simulink model "rov_openloop"  (Simulink 6.0)
settings: Solver=ode45  StartTime=0.0  StopTime=500  RelTol=1e-3
values from neighbouring files (symbols this model uses):
  B = 53400    [npsauv.m]
  Kpdot = -1.0e-3    (= -0.001)    [npsauv.m]
  m = 5454.54/(rho/2*L^3)    (= 0.0732757914251)    [npsauv.m]
  M = r3*(Muw*u*w + Mvv*v^2) +     r4*(Muq*u*q + Mvp*v*p + Mvr*v*r) +     r5*(Mpp*p^2 + Mpr*p*r + Mrr*r^2) -      (xG*W-xB*B)*c1*c2 - (zG*W-zB*B)*s2 +      (Iz-Ix)*p*r + Ixy*q*r - Iyz*p*q - (p^2-r^2)*Ixz +      m*(rho/2*L^3)*(xG*(v*p-u*q) - zG*(w*q-v*r)) + tau5 - rho/2*Cm    [npsauv.m]
  Mqdot = -1.7e-2    (= -0.017)    [npsauv.m]
  Nrdot = -3.4e-3    (= -0.0034)    [npsauv.m]
  W = 53400    [npsauv.m]
  Xudot = -7.6e-3    (= -0.0076)    [npsauv.m]
  Yvdot = -5.5e-2    (= -0.055)    [npsauv.m]
  Zwdot = -2.4e-1    (= -0.24)    [npsauv.m]
undefined symbols (not defined in the file or in its folder): DL, DQ, I, Ma, rg, T, xb, xg, yb, yg, zb, zg
libraries: simulink x8
CloseFcn:
  | rtwprivate ssgensfun ModelCloseRequest openloop
settings Model: LastModifiedBy=c chin

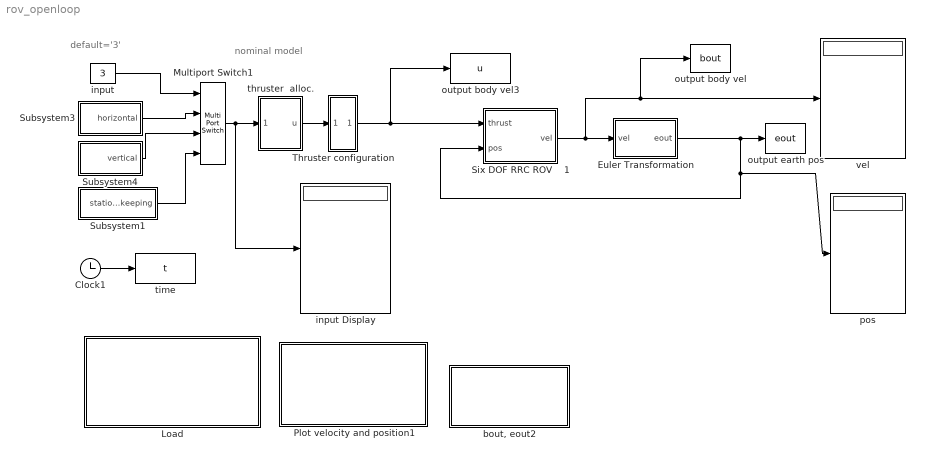
== system rov_openloop ==
  note: nominal model
  note: default='3'
  " Load  " : Subsystem
      settings: OpenFcn=|
      | clc
      | cd c:\Matlab7\toolbox\rov_design_analysis\\mat_file ;
      | load rrcrovf;
      mask Display: disp('Double-click \n to \n Load the\n RRCROV\n parameters')
  " Six DOF RRC ROV    1" : Subsystem
      mask Display:
      | disp('ROV')
      | image(imread('/rov_design_analysis/fig/ROVRRC2.jpg'));
      | color('black');port_label('input',1,'thrust')
      | color('black');port_label('input',2,'pos')
      | color('black');port_label('output',1,'vel')
      | color('black');port_label('output',2,'Inv_MC')
  Clock1 : Clock
      settings: Decimation=10
  Euler Transformation : Subsystem  AncestorBlock=rov_design_analysis/Scope Utilities/Euler Transformation
  Multiport Switch1 : MultiPortSwitch  Inputs=3
  Plot velocity and position1 : Subsystem
      settings: OpenFcn=|
      | clc
      | cd c:\Matlab7\toolbox\rov_design_analysis\\m_file ;
      | run nonlin_resp6
      mask Display: disp('Double-click \n to \n Plot Velocity \n and \n Position')
  Subsystem1 : Subsystem
  Subsystem3 : Subsystem
  Subsystem4 : Subsystem
  Thruster configuration : Subsystem
      mask Display: disp('T')
  "bout, eout2" : Subsystem
      settings: OpenFcn=|
      | clc
      | cd c:\Matlab7\toolbox\rov_design_analysis\\m_file ;
      | figure
      | plot3(eout(:,1), eout(:,2),-eout(:,3))
      | xlabel('x')
      | ylabel('y')
      | zlabel('z')
      | grid on
      mask Display: disp('Plot \n 3D Response')
  input Display : Display
  "input " : Constant  Value=3
  output body vel : ToWorkspace  VariableName=bout  SampleTime=1  SaveFormat=Array
  output body vel3 : ToWorkspace  VariableName=u  SampleTime=1  SaveFormat=Array
  output earth pos : ToWorkspace  VariableName=eout  SampleTime=1  SaveFormat=Array
  pos : Display
  "thruster  alloc.  " : Subsystem
  time : ToWorkspace  VariableName=t  SampleTime=1  SaveFormat=Array
  vel : Display
  wires:
  Thruster configuration/1(output force) -> output body vel3/1, " Six DOF RRC ROV    1"/1("thrust ")
  Clock1/1 -> time/1
  Subsystem4/1(vertical) -> Multiport Switch1/3
  Subsystem3/1(horizontal) -> Multiport Switch1/2
  "input "/1 -> Multiport Switch1/1
  Subsystem1/1(station-keeping) -> Multiport Switch1/4
  Multiport Switch1/1 -> "thruster  alloc.  "/1(ubar_i), input Display/1
  "thruster  alloc.  "/1(u) -> Thruster configuration/1(input velocity)
  Euler Transformation/1(eout) -> output earth pos/1, pos/1, " Six DOF RRC ROV    1"/2("pos ")
  " Six DOF RRC ROV    1"/1(vel) -> Euler Transformation/1(vel), output body vel/1, vel/1

== system rov_openloop/ Load   ==

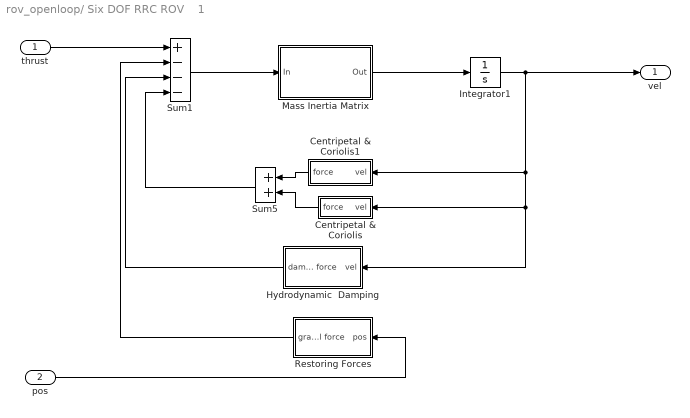
== system rov_openloop/ Six DOF RRC ROV    1 ==
  "thrust " : Inport  Port=1  LatchInput=off
  "pos " : Inport  Port=2  LatchInput=off
  Centripetal & Coriolis : Subsystem  Orientation=left  AncestorBlock=rov_design_analysis/ROV Models/1. Six DOF RRC ROV II/Centripetal & Coriolis
      mask Display: disp('C')
  Centripetal & Coriolis1 : Subsystem  Orientation=left
      mask Display: disp('CA')
  Hydrodynamic  Damping : Subsystem  Orientation=left
      mask Display: disp('Hydrodynamic \nDamping')
  Integrator1 : Integrator
  Mass Inertia Matrix : Subsystem
      mask Display: disp('inv(MRB+MA)')
  Restoring Forces : Subsystem  Orientation=left
      mask Display: disp('Restoring\nForce')
  Sum1 : Sum  Inputs=+---  SaturateOnIntegerOverflow=on  InputSameDT=on
  Sum5 : Sum  Orientation=left  SaturateOnIntegerOverflow=on  InputSameDT=on
  vel : Outport
  wires:
  Restoring Forces/1(gravitational force) -> Sum1/2
  Hydrodynamic  Damping/1(damping force) -> Sum1/3
  "thrust "/1 -> Sum1/1
  Sum1/1 -> Mass Inertia Matrix/1(In)
  Integrator1/1 -> vel/1, Centripetal & Coriolis/1(vel), Hydrodynamic  Damping/1(vel), Centripetal & Coriolis1/1(vel)
  "pos "/1 -> Restoring Forces/1(pos)
  Mass Inertia Matrix/1(Out) -> Integrator1/1
  Centripetal & Coriolis1/1(force) -> Sum5/1
  Centripetal & Coriolis/1(force) -> Sum5/2
  Sum5/1 -> Sum1/4

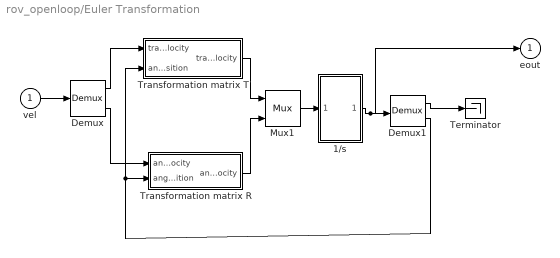
== system rov_openloop/Euler Transformation ==
  vel : Inport  Port=1  LatchInput=off
  1/s : Subsystem
  Demux : Demux  Outputs=2
  Demux1 : Demux  Outputs=2
  Mux1 : Mux  Inputs=2
  Terminator : Terminator
  Transformation matrix R : Subsystem
      mask Display: disp('Transformation R')
  Transformation matrix T : Subsystem
      mask Display: disp('Transformation T')
  eout : Outport  InitialOutput=0
  wires:
  Mux1/1 -> 1/s/1(In1)
  1/s/1(Out1) -> Demux1/1, eout/1
  Demux/2 -> Transformation matrix R/1(angular body  velocity)
  Demux/1 -> Transformation matrix T/1(translational body velocity)
  vel/1 -> Demux/1
  Demux1/2 -> Transformation matrix T/2(angular position), Transformation matrix R/2(angular position)
  Transformation matrix R/1(angular earth velocity) -> Mux1/2
  Transformation matrix T/1(translational earth velocity) -> Mux1/1
  Demux1/1 -> Terminator/1

== system rov_openloop/Plot velocity and position1 ==

== system rov_openloop/Subsystem1 ==
  Mux1 : Mux
  uc{1..4} (4 alike) : Step  Time=0  SampleTime=0
  station-keeping : Outport
  wires:
  uc2/1 -> Mux1/2
  uc1/1 -> Mux1/1
  uc3/1 -> Mux1/3
  uc4/1 -> Mux1/4
  Mux1/1 -> station-keeping/1

== system rov_openloop/Subsystem3 ==
  Mux1 : Mux
  u1 : Step  Time=0  SampleTime=0
  u2 : Step  Time=0  SampleTime=0
  u3 : Step  Time=0  After=0  SampleTime=0
  u4 : Step  Time=0  After=0  SampleTime=0
  horizontal : Outport
  wires:
  u2/1 -> Mux1/2
  u1/1 -> Mux1/1
  u3/1 -> Mux1/3
  Mux1/1 -> horizontal/1
  u4/1 -> Mux1/4

== system rov_openloop/Subsystem4 ==
  Mux1 : Mux
  u1 : Step  Time=0  After=0  SampleTime=0
  u2 : Step  Time=0  After=0  SampleTime=0
  u3 : Step  Time=0  SampleTime=0
  u4 : Step  Time=0  SampleTime=0
  vertical : Outport
  wires:
  u2/1 -> Mux1/2
  u1/1 -> Mux1/1
  u3/1 -> Mux1/3
  u4/1 -> Mux1/4
  Mux1/1 -> vertical/1

== system rov_openloop/Thruster configuration ==
  input velocity : Inport  Orientation=up  Port=1  LatchInput=off
  Thruster Matrix : Gain  Gain=T  Multiplication=Matrix(K*u)  SaturateOnIntegerOverflow=on
  output force : Outport  InitialOutput=0
  wires:
  input velocity/1 -> Thruster Matrix/1
  Thruster Matrix/1 -> output force/1

== system rov_openloop/bout, eout2 ==

== system rov_openloop/thruster  alloc.   ==
  ubar_i : Inport  Port=1  LatchInput=off
  " input" : Constant  Value=[ 1 1 1 1]'
  thruster  allocation control1 : Subsystem  AncestorBlock=|
      | rov_design_analysis/ROV Controller
      | Design
      | Applications/1. Heading autopilot/thruster 
      | allocation control
  u : Outport
  wires:
  ubar_i/1 -> thruster  allocation control1/1(vel)
  " input"/1 -> thruster  allocation control1/2(on/off)
  thruster  allocation control1/1(volt) -> u/1

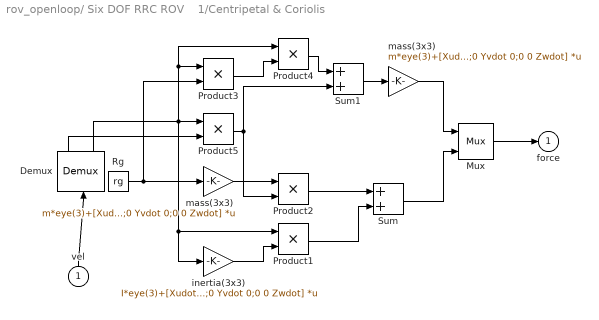
== system rov_openloop/ Six DOF RRC ROV    1/Centripetal & Coriolis ==
  vel : Inport  Orientation=up  Port=1  LatchInput=off
  Demux : Demux  Orientation=up  Outputs=2
  Mux : Mux  Inputs=2
  Product{1..5} (5 alike) : Product  SaturateOnIntegerOverflow=on  RndMeth=Zero  InputSameDT=on
  Rg : Constant  Value=rg
  Sum : Sum  SaturateOnIntegerOverflow=on  InputSameDT=on
  Sum1 : Sum  SaturateOnIntegerOverflow=on  InputSameDT=on
  inertia(3x3) : Gain  Gain=I*eye(3)+[Xudot 0 0;0 Yvdot 0;0 0 Zwdot]  Multiplication=Matrix(K*u)  SaturateOnIntegerOverflow=on
  "mass(3x3) " : Gain  Gain=m*eye(3)+[Xudot 0 0;0 Yvdot 0;0 0 Zwdot]  Multiplication=Matrix(K*u)  SaturateOnIntegerOverflow=on
  "mass(3x3)   " : Gain  Gain=m*eye(3)+[Xudot 0 0;0 Yvdot 0;0 0 Zwdot]  Multiplication=Matrix(K*u)  SaturateOnIntegerOverflow=on
  force : Outport  InitialOutput=0
  wires:
  Product1/1 -> Sum/2
  "mass(3x3)   "/1 -> Product2/1
  Product2/1 -> Sum/1
  Rg/1 -> Product3/2, "mass(3x3)   "/1
  Product3/1 -> Product4/2
  Product4/1 -> Sum1/1
  Product5/1 -> Product2/2, Sum1/2
  Sum1/1 -> "mass(3x3) "/1
  Demux/2 -> Product5/1, Product3/1, Product4/1, Product1/1, inertia(3x3)/1
  Demux/1 -> Product5/2
  vel/1 -> Demux/1
  inertia(3x3)/1 -> Product1/2
  "mass(3x3) "/1 -> Mux/1
  Sum/1 -> Mux/2
  Mux/1 -> force/1

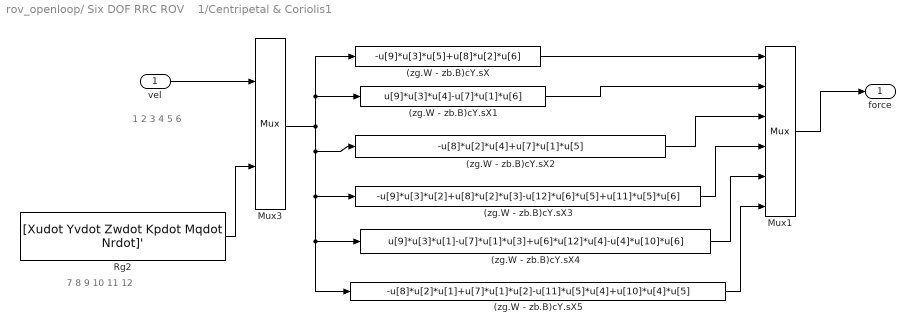
== system rov_openloop/ Six DOF RRC ROV    1/Centripetal & Coriolis1 ==
  note: 7 8 9 10 11 12
  note: 1 2 3 4 5 6
  vel : Inport  Port=1  LatchInput=off
  (zg.W - zb.B)cY.sX : Fcn  Expr=-u[9]*u[3]*u[5]+u[8]*u[2]*u[6]
  (zg.W - zb.B)cY.sX1 : Fcn  Expr=u[9]*u[3]*u[4]-u[7]*u[1]*u[6]
  (zg.W - zb.B)cY.sX2 : Fcn  Expr=-u[8]*u[2]*u[4]+u[7]*u[1]*u[5]
  (zg.W - zb.B)cY.sX3 : Fcn  Expr=-u[9]*u[3]*u[2]+u[8]*u[2]*u[3]-u[12]*u[6]*u[5]+u[11]*u[5]*u[6]
  (zg.W - zb.B)cY.sX4 : Fcn  Expr=u[9]*u[3]*u[1]-u[7]*u[1]*u[3]+u[6]*u[12]*u[4]-u[4]*u[10]*u[6]
  (zg.W - zb.B)cY.sX5 : Fcn  Expr=-u[8]*u[2]*u[1]+u[7]*u[1]*u[2]-u[11]*u[5]*u[4]+u[10]*u[4]*u[5]
  Mux1 : Mux  Inputs=6
  Mux3 : Mux  Inputs=2
  Rg2 : Constant  Value=[Xudot Yvdot Zwdot Kpdot Mqdot Nrdot]'
  force : Outport
  wires:
  Mux1/1 -> force/1
  (zg.W - zb.B)cY.sX/1 -> Mux1/1
  (zg.W - zb.B)cY.sX1/1 -> Mux1/2
  (zg.W - zb.B)cY.sX2/1 -> Mux1/3
  (zg.W - zb.B)cY.sX3/1 -> Mux1/4
  (zg.W - zb.B)cY.sX4/1 -> Mux1/5
  (zg.W - zb.B)cY.sX5/1 -> Mux1/6
  vel/1 -> Mux3/1
  Rg2/1 -> Mux3/2
  Mux3/1 -> (zg.W - zb.B)cY.sX/1, (zg.W - zb.B)cY.sX1/1, (zg.W - zb.B)cY.sX4/1, (zg.W - zb.B)cY.sX5/1, (zg.W - zb.B)cY.sX3/1, (zg.W - zb.B)cY.sX2/1

== system rov_openloop/ Six DOF RRC ROV    1/Hydrodynamic  Damping ==
  vel : Inport  Port=1  LatchInput=off
  D linear : Gain  Gain=-diag(DL)  SaturateOnIntegerOverflow=on
  D quadratic : Gain  Gain=-diag(DQ)  SaturateOnIntegerOverflow=on
  Product : Product  SaturateOnIntegerOverflow=on  RndMeth=Zero  InputSameDT=on
  Sum2 : Sum  SaturateOnIntegerOverflow=on  InputSameDT=on
  |u| : Abs  SaturateOnIntegerOverflow=on
  damping force : Outport  InitialOutput=0
  wires:
  vel/1 -> D linear/1, Product/1, |u|/1
  Product/1 -> D quadratic/1
  |u|/1 -> Product/2
  D quadratic/1 -> Sum2/1
  D linear/1 -> Sum2/2
  Sum2/1 -> damping force/1

== system rov_openloop/ Six DOF RRC ROV    1/Mass Inertia Matrix ==
  In : Inport  Port=1  LatchInput=off
  inverse M : Gain  Gain=inv(M+Ma)  Multiplication=Matrix(K*u)  SaturateOnIntegerOverflow=on
  Out : Outport
  wires:
  inverse M/1 -> Out/1
  In/1 -> inverse M/1

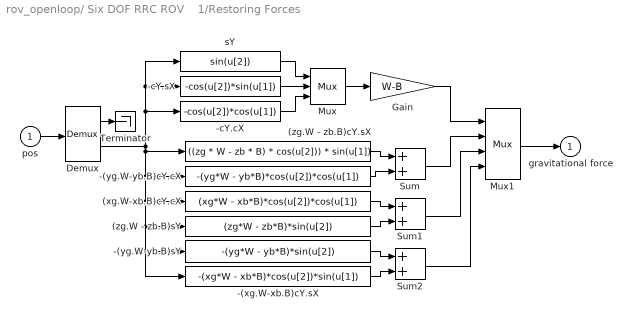
== system rov_openloop/ Six DOF RRC ROV    1/Restoring Forces ==
  pos : Inport  Port=1  LatchInput=off
  (xg.W-xb.B)cY.cX : Fcn  Expr=(xg*W - xb*B)*cos(u[2])*cos(u[1])
  (zg.W - zb.B)cY.sX : Fcn  Expr=((zg * W - zb * B) * cos(u[2])) * sin(u[1])
  (zg.W - zb.B)sY : Fcn  Expr=(zg*W - zb*B)*sin(u[2])
  -(xg.W-xb.B)cY.sX : Fcn  Expr=-(xg*W - xb*B)*cos(u[2])*sin(u[1])
  -(yg.W-yb.B)cY.cX : Fcn  Expr=-(yg*W - yb*B)*cos(u[2])*cos(u[1])
  -(yg.W-yb.B)sY : Fcn  Expr=-(yg*W - yb*B)*sin(u[2])
  -cY.cX : Fcn  Expr=-cos(u[2])*cos(u[1])
  -cY.sX : Fcn  Expr=-cos(u[2])*sin(u[1])
  Demux : Demux  Outputs=2
  Gain : Gain  Gain=W-B  SaturateOnIntegerOverflow=on
  Mux : Mux  Inputs=3
  Mux1 : Mux
  Sum : Sum  SaturateOnIntegerOverflow=on  InputSameDT=on
  Sum1 : Sum  SaturateOnIntegerOverflow=on  InputSameDT=on
  Sum2 : Sum  SaturateOnIntegerOverflow=on  InputSameDT=on
  Terminator : Terminator
  sY : Fcn  Expr=sin(u[2])
  gravitational force : Outport  InitialOutput=0
  wires:
  Sum2/1 -> Mux1/4
  -(yg.W-yb.B)sY/1 -> Sum2/1
  -(xg.W-xb.B)cY.sX/1 -> Sum2/2
  Sum1/1 -> Mux1/3
  (xg.W-xb.B)cY.cX/1 -> Sum1/1
  (zg.W - zb.B)sY/1 -> Sum1/2
  Sum/1 -> Mux1/2
  (zg.W - zb.B)cY.sX/1 -> Sum/1
  -(yg.W-yb.B)cY.cX/1 -> Sum/2
  Gain/1 -> Mux1/1
  Mux/1 -> Gain/1
  -cY.cX/1 -> Mux/3
  -cY.sX/1 -> Mux/2
  sY/1 -> Mux/1
  Mux1/1 -> gravitational force/1
  Demux/2 -> -(xg.W-xb.B)cY.sX/1, -(yg.W-yb.B)sY/1, (zg.W - zb.B)sY/1, (xg.W-xb.B)cY.cX/1, -(yg.W-yb.B)cY.cX/1, (zg.W - zb.B)cY.sX/1, sY/1, -cY.sX/1, -cY.cX/1
  Demux/1 -> Terminator/1
  pos/1 -> Demux/1

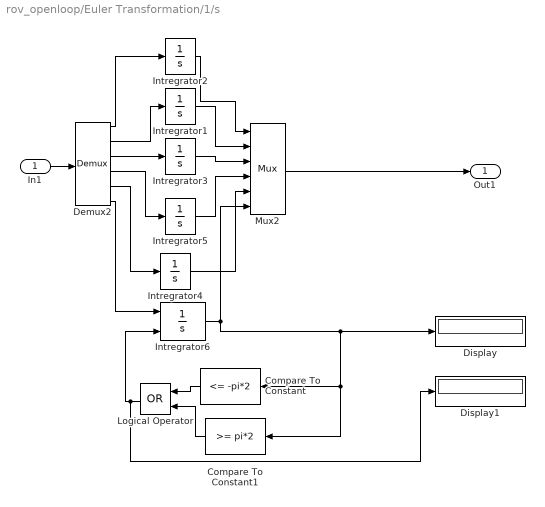
== system rov_openloop/Euler Transformation/1/s ==
  In1 : Inport  Port=1  LatchInput=off
  Compare To Constant : simulink/Logic and Bit Operations/Compare To Constant  Orientation=left  relop=<=  const=-pi*2  LogicOutDataTypeMode=boolean
  Compare To Constant1 : simulink/Logic and Bit Operations/Compare To Constant  Orientation=left  relop=>=  const=pi*2  LogicOutDataTypeMode=boolean
  Demux2 : Demux  Outputs=6
  Display : Display
  Display1 : Display
  Intregrator{1..5} (5 alike) : Integrator
  Intregrator6 : Integrator  ExternalReset=rising  InitialCondition=0.5
  Logical Operator : Logic  Orientation=left  Operator=OR  AllPortsSameDT=off  OutDataTypeMode=Boolean
  Mux2 : Mux  Inputs=6
  Out1 : Outport
  wires:
  Demux2/1 -> Intregrator2/1
  Demux2/2 -> Intregrator1/1
  Demux2/3 -> Intregrator3/1
  Demux2/4 -> Intregrator5/1
  Demux2/5 -> Intregrator4/1
  Intregrator2/1 -> Mux2/1
  Intregrator1/1 -> Mux2/2
  Intregrator3/1 -> Mux2/3
  Intregrator5/1 -> Mux2/4
  In1/1 -> Demux2/1
  Mux2/1 -> Out1/1
  Intregrator4/1 -> Mux2/5
  Demux2/6 -> Intregrator6/1
  Logical Operator/1 -> Intregrator6/2, Display1/1
  Compare To Constant1/1 -> Logical Operator/2
  Compare To Constant/1 -> Logical Operator/1
  Intregrator6/1 -> Display/1, Compare To Constant/1, Compare To Constant1/1, Mux2/6

== system rov_openloop/Euler Transformation/Transformation matrix R ==
  angular body  velocity : Inport  Port=1  LatchInput=off
  angular position : Inport  Port=2  LatchInput=off
  Mux : Mux  Inputs=3
  Row1 of T : Subsystem
      mask Display: disp('Row 1')
  Row2 of T : Subsystem
      mask Display: disp('Row 2')
  Row3 of T : Subsystem
      mask Display: disp('Row 3')
  angular earth velocity : Outport
  wires:
  angular position/1 -> Row3 of T/2(angular position), Row1 of T/2(angular position), Row2 of T/2(angular position)
  Mux/1 -> angular earth velocity/1
  Row3 of T/1(angular earth velocity (row 3)) -> Mux/3
  Row2 of T/1(angular earth velocity (row 2)) -> Mux/2
  Row1 of T/1(angular earth velocity (row 1)) -> Mux/1
  angular body  velocity/1 -> Row3 of T/1("angular body velocity "), Row2 of T/1("angular body velocity "), Row1 of T/1(angular body  velocity)

== system rov_openloop/Euler Transformation/Transformation matrix T ==
  translational body velocity : Inport  Port=1  LatchInput=off
  angular position : Inport  Port=2  LatchInput=off
  Mux : Mux  Inputs=3
  Row1 of R : Subsystem
      mask Display: disp('Row 1')
  Row2 of R : Subsystem
      mask Display: disp('Row 2')
  Row3 of R : Subsystem
      mask Display: disp('Row 3')
  translational earth velocity : Outport  InitialOutput=0
  wires:
  Mux/1 -> translational earth velocity/1
  Row3 of R/1(translational earth velocity (row 3)) -> Mux/3
  Row2 of R/1(translational earth velocity (row 2)) -> Mux/2
  Row1 of R/1(translational earth velocity (row 1)) -> Mux/1
  angular position/1 -> Row3 of R/2(angular position), Row1 of R/2(angular position), Row2 of R/2(angular position)
  translational body velocity/1 -> Row1 of R/1(translational body velocity), Row2 of R/1(translational body velocity), Row3 of R/1(translational body velocity)

== system rov_openloop/thruster  alloc.  /thruster  allocation control1 ==
  vel : Inport  Orientation=down  Port=1  LatchInput=off
  on/off : Inport  Port=2  LatchInput=off
  "thruster allocation " : Subsystem
  volt : Outport
  wires:
  vel/1 -> "thruster allocation "/1(vel)
  on/off/1 -> "thruster allocation "/2(on/off)
  "thruster allocation "/1(volt) -> volt/1

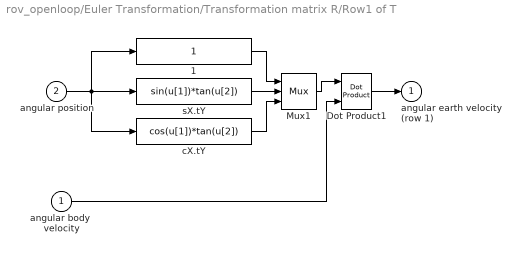
== system rov_openloop/Euler Transformation/Transformation matrix R/Row1 of T ==
  angular body  velocity : Inport  Port=1  LatchInput=off
  angular position : Inport  Port=2  LatchInput=off
  1 : Fcn  Expr=1
  Dot Product1 : simulink/Math Operations/Dot Product  InputSameDT=on  OutDataType=sfix(16)  OutScaling=2^-10  DoSatur=off
  Mux1 : Mux  Inputs=3
  cX.tY : Fcn  Expr=cos(u[1])*tan(u[2])
  sX.tY : Fcn  Expr=sin(u[1])*tan(u[2])
  angular earth velocity (row 1) : Outport
  wires:
  Dot Product1/1 -> angular earth velocity (row 1)/1
  angular body  velocity/1 -> Dot Product1/2
  Mux1/1 -> Dot Product1/1
  cX.tY/1 -> Mux1/3
  sX.tY/1 -> Mux1/2
  1/1 -> Mux1/1
  angular position/1 -> cX.tY/1, sX.tY/1, 1/1

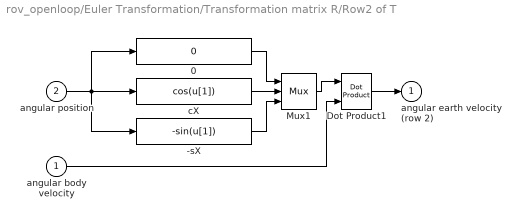
== system rov_openloop/Euler Transformation/Transformation matrix R/Row2 of T ==
  "angular body velocity " : Inport  Port=1  LatchInput=off
  angular position : Inport  Port=2  LatchInput=off
  -sX : Fcn  Expr=-sin(u[1])
  0 : Fcn  Expr=0
  Dot Product1 : simulink/Math Operations/Dot Product  InputSameDT=on  OutDataType=sfix(16)  OutScaling=2^-10  DoSatur=off
  Mux1 : Mux  Inputs=3
  cX : Fcn  Expr=cos(u[1])
  angular earth velocity (row 2) : Outport
  wires:
  Dot Product1/1 -> angular earth velocity (row 2)/1
  "angular body velocity "/1 -> Dot Product1/2
  Mux1/1 -> Dot Product1/1
  -sX/1 -> Mux1/3
  cX/1 -> Mux1/2
  0/1 -> Mux1/1
  angular position/1 -> -sX/1, cX/1, 0/1

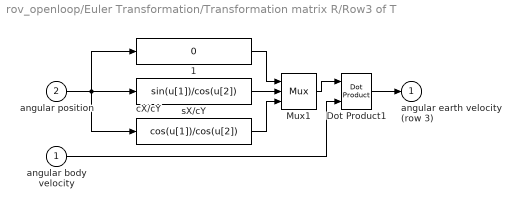
== system rov_openloop/Euler Transformation/Transformation matrix R/Row3 of T ==
  "angular body velocity " : Inport  Port=1  LatchInput=off
  angular position : Inport  Port=2  LatchInput=off
  1 : Fcn  Expr=0
  Dot Product1 : simulink/Math Operations/Dot Product  InputSameDT=on  OutDataType=sfix(16)  OutScaling=2^-10  DoSatur=off
  Mux1 : Mux  Inputs=3
  cX/cY : Fcn  Expr=cos(u[1])/cos(u[2])
  sX/cY : Fcn  Expr=sin(u[1])/cos(u[2])
  angular earth velocity (row 3) : Outport
  wires:
  Dot Product1/1 -> angular earth velocity (row 3)/1
  "angular body velocity "/1 -> Dot Product1/2
  Mux1/1 -> Dot Product1/1
  cX/cY/1 -> Mux1/3
  sX/cY/1 -> Mux1/2
  1/1 -> Mux1/1
  angular position/1 -> cX/cY/1, sX/cY/1, 1/1

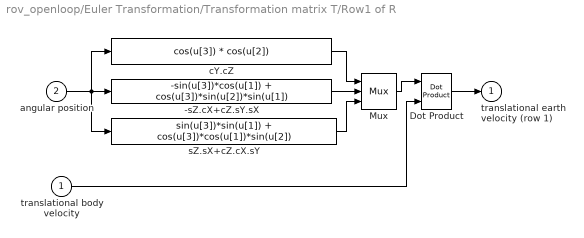
== system rov_openloop/Euler Transformation/Transformation matrix T/Row1 of R ==
  translational body velocity : Inport  Port=1  LatchInput=off
  angular position : Inport  Port=2  LatchInput=off
  -sZ.cX+cZ.sY.sX : Fcn  Expr=-sin(u[3])*cos(u[1]) + cos(u[3])*sin(u[2])*sin(u[1])
  Dot Product : simulink/Math Operations/Dot Product  InputSameDT=on  OutDataType=sfix(16)  OutScaling=2^-10  DoSatur=off
  Mux : Mux  Inputs=3
  cY.cZ : Fcn  Expr=cos(u[3]) * cos(u[2])
  sZ.sX+cZ.cX.sY : Fcn  Expr=sin(u[3])*sin(u[1]) + cos(u[3])*cos(u[1])*sin(u[2])
  translational earth velocity (row 1) : Outport
  wires:
  Dot Product/1 -> translational earth velocity (row 1)/1
  translational body velocity/1 -> Dot Product/2
  Mux/1 -> Dot Product/1
  sZ.sX+cZ.cX.sY/1 -> Mux/3
  -sZ.cX+cZ.sY.sX/1 -> Mux/2
  cY.cZ/1 -> Mux/1
  angular position/1 -> sZ.sX+cZ.cX.sY/1, -sZ.cX+cZ.sY.sX/1, cY.cZ/1

== system rov_openloop/Euler Transformation/Transformation matrix T/Row2 of R ==
  translational body velocity : Inport  Port=1  LatchInput=off
  angular position : Inport  Port=2  LatchInput=off
  -cZ.sX+sY.sZ.cX : Fcn  Expr=-cos(u[3])*sin(u[1]) + sin(u[2])*sin(u[3])*cos(u[1])
  Dot Product1 : simulink/Math Operations/Dot Product  InputSameDT=on  OutDataType=sfix(16)  OutScaling=2^-10  DoSatur=off
  Mux1 : Mux  Inputs=3
  cY.sZ : Fcn  Expr=sin(u[3]) * cos(u[2])
  cZ.cX+sX.sY.sZ : Fcn  Expr=cos(u[3])*cos(u[1]) + sin(u[1])*sin(u[2])*sin(u[3])
  translational earth velocity (row 2) : Outport
  wires:
  Dot Product1/1 -> translational earth velocity (row 2)/1
  translational body velocity/1 -> Dot Product1/2
  Mux1/1 -> Dot Product1/1
  -cZ.sX+sY.sZ.cX/1 -> Mux1/3
  cZ.cX+sX.sY.sZ/1 -> Mux1/2
  cY.sZ/1 -> Mux1/1
  angular position/1 -> -cZ.sX+sY.sZ.cX/1, cZ.cX+sX.sY.sZ/1, cY.sZ/1

== system rov_openloop/Euler Transformation/Transformation matrix T/Row3 of R ==
  translational body velocity : Inport  Port=1  LatchInput=off
  angular position : Inport  Port=2  LatchInput=off
  -sY : Fcn  Expr=-sin(u[2])
  Dot Product1 : simulink/Math Operations/Dot Product  InputSameDT=on  OutDataType=sfix(16)  OutScaling=2^-10  DoSatur=off
  Mux1 : Mux  Inputs=3
  cY.cX : Fcn  Expr=cos(u[2])*cos(u[1])
  cY.sX : Fcn  Expr=cos(u[2])*sin(u[1])
  translational earth velocity (row 3) : Outport  InitialOutput=0
  wires:
  Dot Product1/1 -> translational earth velocity (row 3)/1
  translational body velocity/1 -> Dot Product1/2
  Mux1/1 -> Dot Product1/1
  cY.cX/1 -> Mux1/3
  cY.sX/1 -> Mux1/2
  -sY/1 -> Mux1/1
  angular position/1 -> cY.cX/1, cY.sX/1, -sY/1

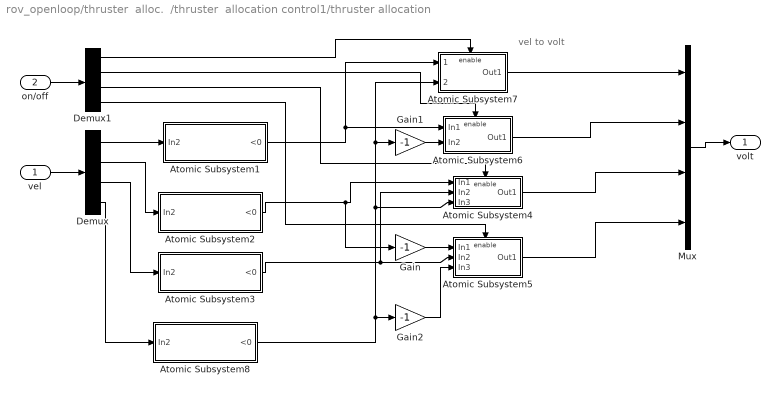
== system rov_openloop/thruster  alloc.  /thruster  allocation control1/thruster allocation  ==
  note: vel to volt
  vel : Inport  Port=1  LatchInput=off
  on/off : Inport  Port=2  LatchInput=off
  Atomic Subsystem1 : Subsystem  TreatAsAtomicUnit=on
      mask Display: disp('check x >0, send \n signal to thrusters ')
  Atomic Subsystem2 : Subsystem  TreatAsAtomicUnit=on
      mask Display: disp('check y >0, send \n signal to thrusters ')
  Atomic Subsystem3 : Subsystem  TreatAsAtomicUnit=on
      mask Display: disp('check z >0, send \n signal to thrusters ')
  Atomic Subsystem4 : Subsystem  TreatAsAtomicUnit=on
      mask Display: disp('activate T3')
  Atomic Subsystem5 : Subsystem  TreatAsAtomicUnit=on
      mask Display: disp('activate T4')
  Atomic Subsystem6 : Subsystem  TreatAsAtomicUnit=on
      mask Display: disp('activate T2')
  Atomic Subsystem7 : Subsystem  TreatAsAtomicUnit=on
      mask Display: disp('activate T1')
  Atomic Subsystem8 : Subsystem  TreatAsAtomicUnit=on
      mask Display: disp('check yaw >0, send \n signal to thrusters ')
  Demux : Demux
  Demux1 : Demux
  Gain : Gain  Gain=-1
  Gain1 : Gain  Gain=-1
  Gain2 : Gain  Gain=-1
  Mux : Mux
  volt : Outport
  wires:
  Demux/1 -> Atomic Subsystem1/1(In2)
  Demux/2 -> Atomic Subsystem2/1(In2)
  Demux/3 -> Atomic Subsystem3/1(In2)
  Atomic Subsystem7/1(Out1) -> Mux/1
  vel/1 -> Demux/1
  Demux/4 -> Atomic Subsystem8/1(In2)
  on/off/1 -> Demux1/1
  Mux/1 -> volt/1
  Atomic Subsystem6/1(Out1) -> Mux/2
  Atomic Subsystem4/1(Out1) -> Mux/3
  Atomic Subsystem5/1(Out1) -> Mux/4
  Atomic Subsystem1/1(<0) -> Atomic Subsystem7/1(1), Atomic Subsystem6/1(In1)
  Atomic Subsystem2/1(<0) -> Atomic Subsystem4/1(In1), Gain/1
  Atomic Subsystem3/1(<0) -> Atomic Subsystem4/2(In2), Atomic Subsystem5/2(In2)
  Gain/1 -> Atomic Subsystem5/1(In1)
  Atomic Subsystem8/1(<0) -> Atomic Subsystem7/2(2), Gain1/1, Atomic Subsystem4/3(In3), Gain2/1
  Gain1/1 -> Atomic Subsystem6/2(In2)
  Gain2/1 -> Atomic Subsystem5/3(In3)
  Demux1/1 -> Atomic Subsystem7/Enable
  Demux1/2 -> Atomic Subsystem6/Enable
  Demux1/3 -> Atomic Subsystem4/Enable
  Demux1/4 -> Atomic Subsystem5/Enable

== system rov_openloop/thruster  alloc.  /thruster  allocation control1/thruster allocation /Atomic Subsystem1 ==
  In2 : Inport  Port=1  LatchInput=off
  Abs : Abs
  Product1 : Product  OutDataTypeMode=double  SaturateOnIntegerOverflow=on  RndMeth=Zero
  Product5 : Product  OutDataTypeMode=double  SaturateOnIntegerOverflow=on  RndMeth=Zero
  Sign1 : Signum
  Switch1 : Switch  Threshold=1  SaturateOnIntegerOverflow=on  InputSameDT=on
  <0 : Outport
  wires:
  Sign1/1 -> Product1/2, Product5/1, Switch1/2
  Product1/1 -> Switch1/1
  Product5/1 -> Switch1/3
  Switch1/1 -> <0/1
  In2/1 -> Sign1/1, Product1/1, Abs/1
  Abs/1 -> Product5/2

== system rov_openloop/thruster  alloc.  /thruster  allocation control1/thruster allocation /Atomic Subsystem2 ==
  In2 : Inport  Port=1  LatchInput=off
  Abs : Abs
  Product1 : Product  OutDataTypeMode=double  SaturateOnIntegerOverflow=on  RndMeth=Zero
  Product5 : Product  OutDataTypeMode=double  SaturateOnIntegerOverflow=on  RndMeth=Zero
  Sign1 : Signum
  Switch1 : Switch  Threshold=1  SaturateOnIntegerOverflow=on  InputSameDT=on
  <0 : Outport
  wires:
  In2/1 -> Sign1/1, Product1/1, Abs/1
  Sign1/1 -> Switch1/2, Product1/2, Product5/1
  Product1/1 -> Switch1/1
  Product5/1 -> Switch1/3
  Switch1/1 -> <0/1
  Abs/1 -> Product5/2

== system rov_openloop/thruster  alloc.  /thruster  allocation control1/thruster allocation /Atomic Subsystem3 ==
  In2 : Inport  Port=1  LatchInput=off
  Abs : Abs
  Product1 : Product  OutDataTypeMode=double  SaturateOnIntegerOverflow=on  RndMeth=Zero
  Product5 : Product  OutDataTypeMode=double  SaturateOnIntegerOverflow=on  RndMeth=Zero
  Sign1 : Signum
  Switch1 : Switch  Threshold=1  SaturateOnIntegerOverflow=on  InputSameDT=on
  <0 : Outport
  wires:
  Sign1/1 -> Switch1/2, Product1/2, Product5/1
  Product1/1 -> Switch1/1
  Product5/1 -> Switch1/3
  Switch1/1 -> <0/1
  In2/1 -> Sign1/1, Product1/1, Abs/1
  Abs/1 -> Product5/2

== system rov_openloop/thruster  alloc.  /thruster  allocation control1/thruster allocation /Atomic Subsystem4 ==
  In1 : Inport  Port=1  LatchInput=off
  In2 : Inport  Port=2  LatchInput=off
  In3 : Inport  Port=3  LatchInput=off
  Enable : EnablePort
  Subtract : Sum  Inputs=+++  OutScaling=2^-10
  Out1 : Outport
  wires:
  In1/1 -> Subtract/1
  In2/1 -> Subtract/2
  In3/1 -> Subtract/3
  Subtract/1 -> Out1/1

== system rov_openloop/thruster  alloc.  /thruster  allocation control1/thruster allocation /Atomic Subsystem5 ==
  In1 : Inport  Port=1  LatchInput=off
  In2 : Inport  Port=2  LatchInput=off
  In3 : Inport  Port=3  LatchInput=off
  Enable : EnablePort
  Subtract : Sum  Inputs=+++  OutScaling=2^-10
  Out1 : Outport
  wires:
  In1/1 -> Subtract/1
  In2/1 -> Subtract/2
  In3/1 -> Subtract/3
  Subtract/1 -> Out1/1

== system rov_openloop/thruster  alloc.  /thruster  allocation control1/thruster allocation /Atomic Subsystem6 ==
  In1 : Inport  Port=1  LatchInput=off
  In2 : Inport  Port=2  LatchInput=off
  Enable : EnablePort
  Subtract : Sum  OutScaling=2^-10
  Out1 : Outport
  wires:
  In1/1 -> Subtract/1
  In2/1 -> Subtract/2
  Subtract/1 -> Out1/1

== system rov_openloop/thruster  alloc.  /thruster  allocation control1/thruster allocation /Atomic Subsystem7 ==
  1 : Inport  Port=1  LatchInput=off
  2 : Inport  Port=2  LatchInput=off
  Enable : EnablePort
  Subtract : Sum  OutScaling=2^-10
  Out1 : Outport
  wires:
  1/1 -> Subtract/1
  2/1 -> Subtract/2
  Subtract/1 -> Out1/1

== system rov_openloop/thruster  alloc.  /thruster  allocation control1/thruster allocation /Atomic Subsystem8 ==
  In2 : Inport  Port=1  LatchInput=off
  Abs : Abs
  Product1 : Product  OutDataTypeMode=double  SaturateOnIntegerOverflow=on  RndMeth=Zero
  Product5 : Product  OutDataTypeMode=double  SaturateOnIntegerOverflow=on  RndMeth=Zero
  Sign1 : Signum
  Switch1 : Switch  Threshold=1  SaturateOnIntegerOverflow=on  InputSameDT=on
  <0 : Outport
  wires:
  In2/1 -> Sign1/1, Product1/1, Abs/1
  Sign1/1 -> Switch1/2, Product1/2, Product5/1
  Product1/1 -> Switch1/1
  Product5/1 -> Switch1/3
  Switch1/1 -> <0/1
  Abs/1 -> Product5/2
